simulink model "Hunt_crossley_Ident_simpleMCMC"  (Simulink 8.0)
settings: Solver=ode3  StartTime=0.0  StopTime=20  FixedStep=0.001  RelTol=1e-3
libraries: dspstat3 x1
settings Model: Creator=x  LastModifiedBy=x
settings DebuggingCC: FrameProcessingCompatibilityMsg=error
settings CodeAppCC: CustomSymbolStrType=$N$R$M_T  InternalIdentifier=Shortened
settings GRTTargetCC: CodeReplacementLibrary=None  CPPClassGenCompliant=on

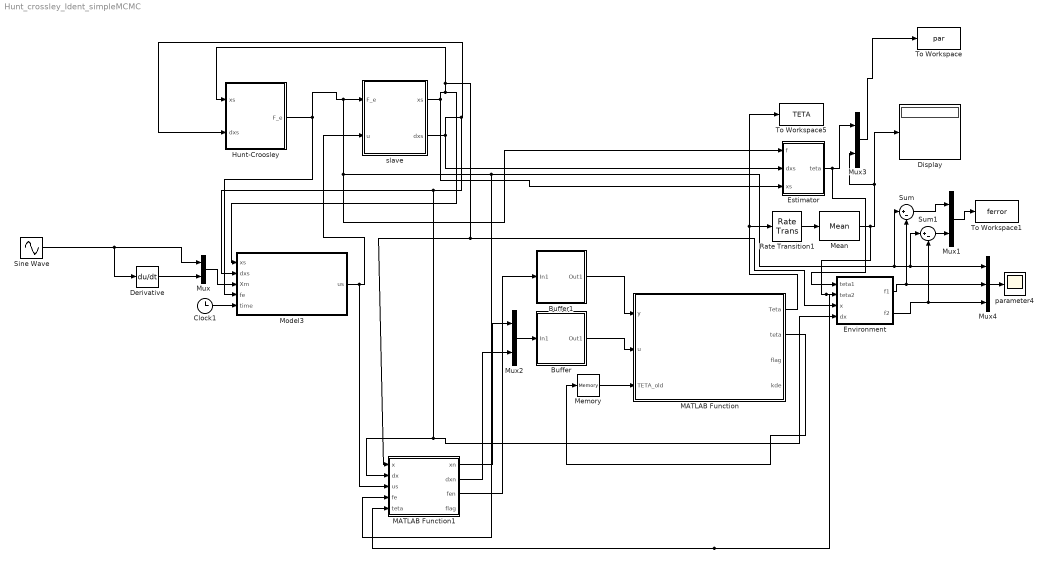
== system Hunt_crossley_Ident_simpleMCMC ==
  Buffer : Subsystem
  Buffer1 : Subsystem
  Clock1 : Clock
  Derivative : Derivative
  Display : Display
  Environment : MATLAB Function  TreatAsAtomicUnit=on
  Estimator : Subsystem
  Hunt-Croosley : Subsystem
  MATLAB Function : MATLAB Function  TreatAsAtomicUnit=on
  MATLAB Function1 : MATLAB Function  TreatAsAtomicUnit=on
  Mean : dspstat3/Mean  run=off  reset_popup=None  InputProcessing=Columns as channels (frame based)  directionMode=Each row  dimension=1  treatSBRowAsCol=on  roiEnable=off  roiType=Rectangles  roiPortion=Entire ROI  roiOutput=Individual statistics for each ROI  roiFlag=off  outputDataTypeStr=Inherit: Same as accumulator  outputLastDataTypeStr=Inherit: Same as accumulator  outputMin=[]  outputMax=[]  roundingMode=Floor  overflowMode=off
  Memory : Memory  X0=[1;1 ;1]*1*ones(1,2000)  InheritSampleTime=on
  Model3 : MATLAB Function  TreatAsAtomicUnit=on
  Mux{,1..3} (4 alike) : Mux  Inputs=2
  Mux4 : Mux  Inputs=3
  Rate Transition1 : RateTransition  OutPortSampleTime=0.001
  Sine Wave : Sin  Bias=0.6  SampleTime=0
  Sum : Sum  Inputs=|+-
  Sum1 : Sum  Inputs=|+-
  To Workspace : ToWorkspace  VariableName=par  SampleTime=-1
  To Workspace1 : ToWorkspace  VariableName=ferror  SampleTime=-1
  To Workspace5 : ToWorkspace  VariableName=TETA  SampleTime=-1
  parameter4 : Scope
  slave : Subsystem
  wires:
  Sine Wave/1 -> Derivative/1, Mux/1
  Clock1/1 -> Model3/5(time)
  Derivative/1 -> Mux/2
  Mux/1 -> Model3/3(Xm)
  Mux2/1 -> Buffer/1(In1)
  MATLAB Function/2(teta) -> Memory/1
  Buffer/1(Out1) -> MATLAB Function/2(u)
  Buffer1/1(Out1) -> MATLAB Function/1(y)
  Rate Transition1/1 -> Mean/1
  Memory/1 -> MATLAB Function/3(TETA_old)
  Mux3/1 -> To Workspace/1
  Estimator/1(teta) -> Environment/1(teta1), Mux3/1
  MATLAB Function1/1(xn) -> Mux2/1
  MATLAB Function1/2(dxn) -> Mux2/2
  slave/2(dxs) -> Model3/2(dxs), Environment/4(dx), MATLAB Function1/2(dx), Hunt-Croosley/2(dxs), Estimator/2(dxs)
  slave/1(xs) -> Model3/1(xs), MATLAB Function1/1(x), Environment/3(x), Hunt-Croosley/1(xs), Estimator/3(xs)
  Model3/1(us) -> slave/2(u), MATLAB Function1/3(us)
  Environment/1(f1) -> Mux4/2, Sum/2
  Mux4/1 -> parameter4/1
  Hunt-Croosley/1(F_e) -> slave/1(F_e), Sum/1, Sum1/1, Mux4/1, MATLAB Function1/4(fe), Estimator/1(f), Model3/4(fe)
  MATLAB Function/1(Teta) -> To Workspace5/1, Rate Transition1/1
  MATLAB Function1/3(fen) -> Buffer1/1(In1)
  Mean/1 -> MATLAB Function1/5(teta), Environment/2(teta2), Mux3/2, Display/1
  Sum/1 -> Mux1/1
  Mux1/1 -> To Workspace1/1
  Environment/2(f2) -> Mux4/3, Sum1/2
  Sum1/1 -> Mux1/2

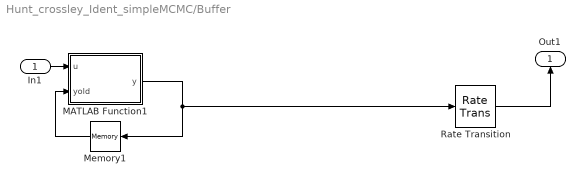
== system Hunt_crossley_Ident_simpleMCMC/Buffer ==
  In1 : Inport
  MATLAB Function1 : MATLAB Function  TreatAsAtomicUnit=on
  Memory1 : Memory  X0=zeros(100,2)  LinearizeMemory=on
  Rate Transition : RateTransition  X0=zeros(200,2)  OutPortSampleTime=0.2
  Out1 : Outport
  wires:
  Rate Transition/1 -> Out1/1
  Memory1/1 -> MATLAB Function1/2(yold)
  In1/1 -> MATLAB Function1/1(u)
  MATLAB Function1/1(y) -> Rate Transition/1, Memory1/1

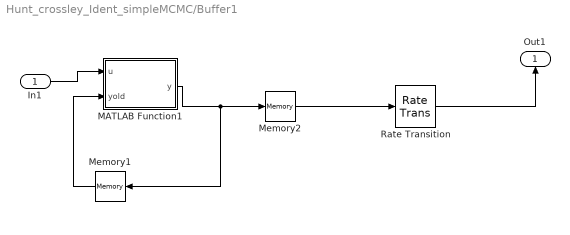
== system Hunt_crossley_Ident_simpleMCMC/Buffer1 ==
  In1 : Inport
  MATLAB Function1 : MATLAB Function  TreatAsAtomicUnit=on
  Memory1 : Memory  X0=zeros(200,1)  LinearizeMemory=on
  Memory2 : Memory  X0=zeros(200,1)  LinearizeMemory=on
  Rate Transition : RateTransition  X0=zeros(200,1)  OutPortSampleTime=0.2
  Out1 : Outport
  wires:
  Memory1/1 -> MATLAB Function1/2(yold)
  Rate Transition/1 -> Out1/1
  MATLAB Function1/1(y) -> Memory2/1, Memory1/1
  Memory2/1 -> Rate Transition/1
  In1/1 -> MATLAB Function1/1(u)

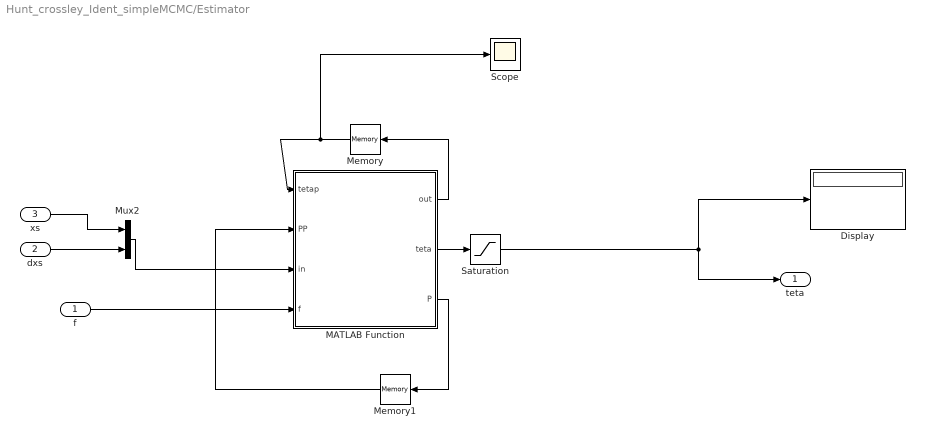
== system Hunt_crossley_Ident_simpleMCMC/Estimator ==
  f : Inport
  dxs : Inport  Port=2
  xs : Inport  Port=3
  Display : Display
  MATLAB Function : MATLAB Function  TreatAsAtomicUnit=on
  Memory : Memory
  Memory1 : Memory
  Mux2 : Mux  Inputs=2
  Saturation : Saturate  UpperLimit=5  LowerLimit=0
  Scope : Scope
  teta : Outport
  wires:
  f/1 -> MATLAB Function/4(f)
  MATLAB Function/1(out) -> Memory/1
  Memory1/1 -> MATLAB Function/2(PP)
  Mux2/1 -> MATLAB Function/3(in)
  Memory/1 -> Scope/1, MATLAB Function/1(tetap)
  xs/1 -> Mux2/1
  dxs/1 -> Mux2/2
  MATLAB Function/3(P) -> Memory1/1
  MATLAB Function/2(teta) -> Saturation/1
  Saturation/1 -> teta/1, Display/1

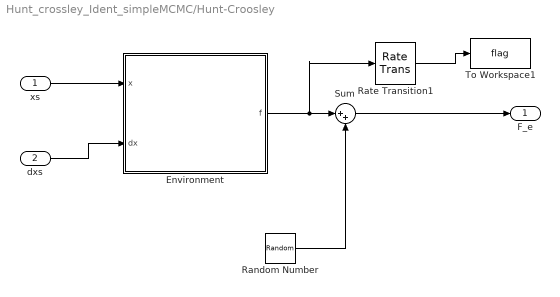
== system Hunt_crossley_Ident_simpleMCMC/Hunt-Croosley ==
  xs : Inport
  dxs : Inport  Port=2
  Environment : MATLAB Function  TreatAsAtomicUnit=on
  Random Number : RandomNumber  Variance=0.01  SampleTime=0.001
  Rate Transition1 : RateTransition  OutPortSampleTime=0.1
  Sum : Sum  Inputs=|++
  To Workspace1 : ToWorkspace  VariableName=flag  SampleTime=-1
  F_e : Outport
  wires:
  xs/1 -> Environment/1(x)
  dxs/1 -> Environment/2(dx)
  Environment/1(f) -> Rate Transition1/1, Sum/1
  Sum/1 -> F_e/1
  Random Number/1 -> Sum/2
  Rate Transition1/1 -> To Workspace1/1

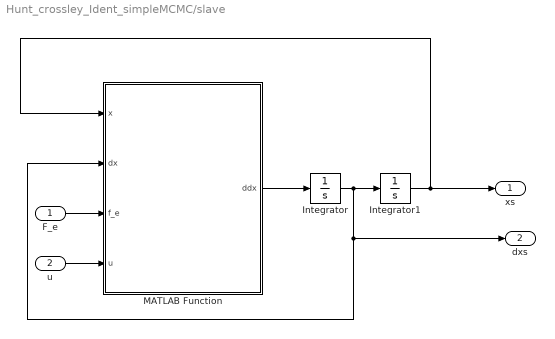
== system Hunt_crossley_Ident_simpleMCMC/slave ==
  F_e : Inport
  u : Inport  Port=2
  Integrator : Integrator
  Integrator1 : Integrator
  MATLAB Function : MATLAB Function  TreatAsAtomicUnit=on
  xs : Outport
  dxs : Outport  Port=2
  wires:
  F_e/1 -> MATLAB Function/3(f_e)
  u/1 -> MATLAB Function/4(u)
  MATLAB Function/1(ddx) -> Integrator/1
  Integrator/1 -> dxs/1, MATLAB Function/2(dx), Integrator1/1
  Integrator1/1 -> xs/1, MATLAB Function/1(x)

== matlab function slave/MATLAB Function ==
  data: x input double; dx input double; f_e input double; u input double; ddx output double
function ddx = fcn(x,dx,f_e,u)
%parameter
ms=0.07; bs=0.05;ks=0.08; 
ms=1; bs=0.5;ks=0.8; 

ddx=ms^-1*(u-f_e-bs*dx-ks*x);

== matlab function MATLAB Function ==
  data: Teta output double; y input double; u input double; TETA_old input double; teta output double; flag output double; kde output double
function [Teta,teta,flag,kde]  = online_mcmc(y,u  ,TETA_old)
coder.extrinsic('ksdensity');
coder.extrinsic('unifrnd');
kde_y=zeros(1,100);
kde_x=zeros(1,100);
kde=zeros(2,100);
n=100;
lambda=0.95;
SampNum=2000;%2000
nac=0;
count = 0;
ParNum = 3;
sigma2_RW = .001;%0.0001
sigma2 = 0.03;   
% preallcoation for speed
epsi=zeros(ParNum, 1);
ye1=0;
flag=0; %noninformative prior
inint_ths=10^22;
inint_ths=0.01;
init_low=1.5;
init_high=4.5;
SampMin=1000;%1000
AccMin=0.5;
npdf=1/sqrt(2*pi*sigma2^2);

ye1_candid = 0;
TETA_old =TETA_old.*0;

%%%%%%%%%%%%%%%%%%%%%%%%%%%% special cases (flag=2)%%%%%%%%%%%%%%%%%%%%%%%%%%%%%%%%%%%
% no environment
for i2 = 1:n
    if (u(i2,1)<0 && u(i2,2)<0 ) || (u(i2,1)<-0.001*sqrt(sigma2)*rand)
        count=count+1*0*(exp(-lambda*(n-i2)))+1;
    end
end
% start up
if min(y)==0 && max(y)==0 
    teta=TETA_old*0;
    flag=2*0;
    
elseif count>0.85*n
    teta=TETA_old*0;
    flag=2*0;
else
 u(:,1)=abs(u(:,1));
%%%%%%%%%%%%%%%%%%%%%%%%%%%% Normal cases (flag!=2)%%%%%%%%%%%%%%%%%%%%%%%%%%%%%%%%%%%
  %--------------------- Initializing -----------------------------------
dummy=0;
teta=[TETA_old(:,2:end), (mean(TETA_old(:,floor(SampNum/2):end)'))'];
for i2 = 1:n
    %ye1(i2) = u(i2,:) * teta(:,end) ;
    dumm=teta(1,end)+teta(2,end)*u(i2,2);
    if dumm <0
        dummy=-inf;
        break;
    end
    ye1 = teta(3,end)*log10(u(i2,1))+log10(dumm) ;
    dummy=log10(npdf*exp(-(exp(-lambda*(n-i2)))*(y(i2) - 10^ye1)^2/sigma2^2))+dummy;
    %dummy = log10(normpdf(y(i2) - ye1(i2), 0, sigma2)) + dummy;
end

if 10^dummy>inint_ths
    prob_teta = dummy;
    
% %%%%%%%%%%%%%%%%%%%% informative prior (flag=1)%%%%%%%%%%%%%%%%%%%%%%%%%%
%     
%     sigma2_RW=0.0008*sigma2_RW;
%  for  k = 1:SampNum
%       
%         %-------------------- Introducing Candidate ---------------------------
% %                          epsi(:,k) = teta(:,k) + normrnd(0,sqrt(sigma2_RW),[size(teta,1),1]);
%                             epsi= teta(:,ceil(rand*ParNum))+sqrt(sigma2_RW)*randn([size(teta,1),1]); 
%                             
% 
%         %-------------------- Evaluating Acceptance ---------------------------
% 
%         % Prior Knowledg
%         if ( epsi(1)>5 ) ||( epsi(1)<0 ) || (epsi(2)> 5) ||(epsi(2)< 0) ||  ( epsi(3) > 2)||(epsi(3)< 1) 
%             prob_epsi = -inf;
%         else
% 
%             ye1_candid = 0;
%             dummy = 0; % Computing Probability of Epsilon Parameter
%             for i2 = 1:n
%                 % ---- Computing candidate probability accordance to noise distribution ----
% 
% %                 ye1_candid(i2) =  u(i2,:) * epsi(:);
%                  dumm= epsi(1)+epsi(2)*u(i2,2);
%                  if dumm<0
%                      dummy=-inf;
%                      break;
%                  end
%                 ye1_candid = epsi(3)*log10(u(i2,1))+log10(dumm) ;
%                 
% 
%                 %dummy = log10(normpdf(y(i2) - ye1_candid(i2), 0,sigma2)) + dummy;
%                 dummy=log10(npdf*exp(-(exp(-lambda*(n-i2)))*(y(i2) - 10^ye1_candid)^2/sigma2^2))+dummy;
% 
%             end
% 
%             prob_epsi = dummy;
% 
%         end
%         alpha = min(1,10^(prob_epsi-prob_teta));
%         z = rand(1,1);
%         
%             if (z < alpha)
%                 teta = [teta(:,2:end), epsi];
%                 prob_teta = prob_epsi;
%                 nac=nac+1;
%             else
%                 teta = [teta(:,2:end), teta(:,end)];
%             end
%             
%             if (k>SampMin && nac <k*AccMin)
%                 break;
%             end
%             if (k==floor(0.75*SampMin) && nac <0.5*k*AccMin)
%                 sigma2_RW=0.1*sigma2_RW;
%             end
%             if (k==0.5*SampMin && nac <0.5*k*AccMin)
%                 sigma2_RW=0.1*sigma2_RW;
%             end
%       
%  end
%    
%    flag=1*0; 
end




%%%%%%%%%%%%%%%%%%%% non informative prior (flag=0)%%%%%%%%%%%%%%%%%%%%%%%%%%

dummy = -inf;
%while (isinf(dummy))
 while (10^dummy<10^22*5e7*100)
    teta(:,1) = unifrnd(init_low,init_high,[ParNum,1]);
    teta(2,1) = unifrnd(1,3);
    teta(3,1) = unifrnd(1,2);
    dummy = 0; % Computing Probability of Previous Sample Parameter
            
   % ye1 = 0; 
            
    for i2 = 1:n

%            ye1(i2) = u(i2,:) * teta(:,1);
            dumm = teta(1,1)+teta(2,1)*u(i2,2);
            if dumm<0
                dummy=-inf;
                break;
            end
           ye1 = teta(3,1)*log10(u(i2,1))+log10(dumm) ;
                    % -------- Computing first step of MCMC accordance to noise type ------
           %dummy = log10(normpdf(y(i2) - ye1(i2), 0, sigma2)) + dummy ;
           dummy=log10(npdf*exp(-(exp(-lambda*(n-i2)))*(y(i2) - 10^ye1)^2/sigma2^2))+dummy;

           if isinf(dummy)
                 break;
           end

    end

    prob_teta = dummy; 
%     count = count + 1
end

for  k = 1:(SampNum-1)
    
    prob_teta = dummy;
      
        %-------------------- Introducing Candidate ---------------------------
                     
               epsi = teta(:,k) +sqrt(sigma2_RW)*randn([size(teta,1),1]);
                      
        %-------------------- Evaluating Acceptance ---------------------------
          % Prior Knowledg
        if ( epsi(1)>5 ) ||( epsi(1)<0 ) || (epsi(2)> 5) ||(epsi(2)< 0) ||  ( epsi(3) > 2)||(epsi(3)< 1) 
            prob_epsi = -inf;
        else

            ye1_candid = 0;
            dummy = 0; % Computing Probability of Epsilon Parameter
            for i2 = 1:n
                % ---- Computing candidate probability accordance to noise distribution ----

%                 ye1_candid(i2) =  u(i2,:) * epsi(:);

                dumm = epsi(1)+epsi(2)*u(i2,2);
            if dumm<0
                dummy=-inf;
                break;
            end
                ye1_candid = epsi(3)*log10(u(i2,1))+log10(dumm) ;

                %dummy = log10(normpdf(y(i2) - ye1_candid(i2), 0,sigma2)) + dummy;
                dummy=log10(npdf*exp(-(exp(-lambda*(n-i2)))*(y(i2) - 10^ye1_candid)^2/sigma2^2))+dummy;

            end

            prob_epsi = dummy;

        end

        alpha = min(1,10^(prob_epsi-prob_teta));
        z = rand(1,1);
        
            if (z < alpha)
                teta(:,k+1) = epsi;
                prob_teta = prob_epsi;
                nac=nac+1;
            else
                teta(:,k+1) = teta(:,k);
            end
            
           % if (k>2*SampMin && nac<0.5*k*AccMin)
           %     break;
           % end
            if (k==floor(1.5*SampMin) && nac <0.5*k*AccMin)
                sigma2_RW=0.5*sigma2_RW;
            end
            if (k==2*SampMin && nac <0.8*k*AccMin)
                sigma2_RW=0.5*sigma2_RW;
            end
end
    
%nac=nac/k;
end


[kde_x,kde_y]=ksdensity(teta(1,500:end));
kde=[kde_x ;kde_y];
%plot(kde_y ,kde_x);
[kde_x,kde_y]=ksdensity(teta(2,500:end));
%%figure(2);
%%plot(kde_y ,kde_x);
%[kde_x,kde_y]=ksdensity(teta(3,500:end));
%figure(3);
%plot(kde_y ,kde_x);
Teta=teta(:,500:end);
end

== matlab function Estimator/MATLAB Function ==
  data: out output double; tetap input double; PP input double; in input double; f input double; teta output double; P output double
function [out, teta, P]= fcn(tetap,   PP,   in,   f)
%parameter
landa=1;
if (in(1)<0.1 || f<0.1)
   out=[1;1;1];
   teta=[0;0;1];
   P=10^3*eye(3,3);
else
phi=[1;in(2);log(in(1))];
L=PP*phi/(landa+phi'*PP*phi);
P=1/landa*(PP-L*phi'*PP);
out=tetap+L*(log(f)-phi'*tetap);
teta=[exp(out(1)); out(2)*exp(out(1));out(3)];
if (P(1,1)>1000)
    P(1,1)=1000;
end
if (P(2,2)>1000)
     P(2,2)=1000;
end
if (P(3,3)>1000)
     P(3,3)=1000;
end
end
end

== matlab function Buffer/MATLAB Function1 ==
  data: u input double; y output double; yold input double
function y = fcn(u,yold)
%#codegen

y = [yold(2:200,:);u'];

== matlab function Hunt-Croosley/Environment ==
  data: x input double; dx input double; f output double
function f= ENV( x,dx )
%   Parameter
K=4;B=2.3; n=1.7;
K=4;B=2.3; n=1.7;

if x<0
    f=0;
else
    f=(x^n)*(K+B*dx);
end

end

== matlab function Buffer1/MATLAB Function1 ==
  data: u input double; y output double; yold input double
function y = fcn(u,yold)
%#codegen

y = [yold(2:200);u];

== matlab function Model3 ==
  data: xs input double; dxs input double; Xm input double; fe input double; us output double; time input double
function us= slave_Impedance_control( xs,dxs,Xm,fe,time )
%   Parameter
ms=1; bs=0.5;ks=0.8; 
jsd=50; bsd=150;ksd=100;
if time==0.001
    us=0;
else
xm=Xm(1);
dxm=Xm(2);
us=-(ms/jsd*bsd)*(dxs-dxm)-(ms/jsd*ksd)*(xs-xm)+(1-0*ms/jsd)*fe+bs*dxs+ks*xs;
end
end

== matlab function MATLAB Function1 ==
  data: x input double; dx input double; us input double; fe input double; xn output double; dxn output double; fen output double; teta input double; flag output double
function [xn,dxn,fen,flag]=prediction(x,dx,us,fe,teta)
%parameter
Ts=0.2;
ms=1; bs=0.5;ks=0.8; 
a2=-ks/ms;
b=1/ms;
a1=-bs/ms;
Ke=teta(1);
Be=teta(2);
n=teta(3);
Ke=4;
Be=2.3;
n=1.7;
Thr=0;
% estimated environment force
if x<0
    feest=0;
else
feest=(Ke+Be*dx)*x^n;
end

if abs(feest-fe)>Thr
%% stage 0: Teta is no valid
% Prediciton horizen
xn=x;
dxn=dx;
fen=fe;
flag=0;

else
%% stage 1:  valid Teta
xn=x+Ts*dx;
dxn=a2/a1*(1-exp(a1*Ts))*x+exp(a1*Ts)*dx-Ts/ms*feest-b/a1*(1-exp(a1*Ts))*us;
if xn<0
    fen=0;
else
fen=(Ke+Be*dxn)*xn^n;
end
flag=1;

end
end

== matlab function Environment ==
  data: teta1 input double; teta2 input double; x input double; dx input double; f1 output double; f2 output double
function [f1,f2]= ENV( teta1,teta2, x,dx )
%   Parameter
K=teta1(1);B=teta1(2); n=teta1(3);

x=abs(x);
 f1=(x^n)*(K+B*dx);
 
 
K=teta2(1);B=teta2(2); n=teta2(3);
 f2=(x^n)*(K+B*dx);
% if x<0
%     f=0;
% else
%     f=(x^n)*(K+B*dx);
% end

end
